simulink library "IOLib"  (R2016b)
settings: Solver=VariableStepAuto  StartTime=0.0  StopTime=10.0  RelTol=1e-3
undefined symbols (not defined in the file): EGPI, EGPO, EVADC
libraries: simulink x3
settings Model: Creator=Administrator  LastModifiedBy=Administrator

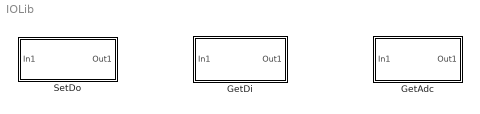
== system IOLib ==
  GetAdc : Subsystem  TreatAsAtomicUnit=on
      settings: OpenFcn=open_system([gcb,'/Enumerated Constant'],'mask');  RTWSystemCode=Inline
      mask Display:
      | tmpx = get_param([gcb,'/Enumerated Constant'],'Value');
      | disp(tmpx);
  GetDi : Subsystem  TreatAsAtomicUnit=on
      settings: OpenFcn=open_system([gcb,'/Enumerated Constant'],'mask');  PermitHierarchicalResolution=None  RTWSystemCode=Inline
      mask Display:
      | tmpx = get_param([gcb,'/Enumerated Constant'],'Value');
      | disp(tmpx);
  SetDo : Subsystem  TreatAsAtomicUnit=on
      settings: OpenFcn=open_system([gcb,'/Enumerated Constant'],'mask');  RTWSystemCode=Inline
      mask Display:
      | tmpx = get_param([gcb,'/Enumerated Constant'],'Value');
      | disp(tmpx);

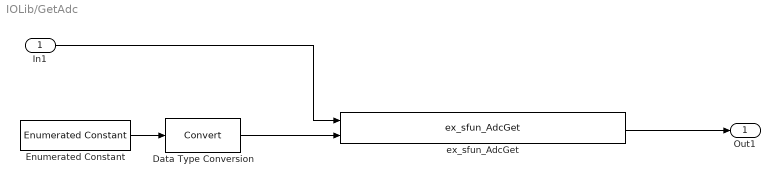
== system IOLib/GetAdc ==
  In1 : Inport
  Data Type Conversion : DataTypeConversion
  Enumerated Constant : simulink/Sources/Enumerated Constant  OutDataTypeStr=Enum: EVADC  Value=EVADC.UBR1  SampleTime=inf
  ex_sfun_AdcGet : S-Function  FunctionName=ex_sfun_AdcGet  SFunctionDeploymentMode=off  EnableBusSupport=off  mask(Legacy Function){SFunctionSpec=void AdcGetShell(uint16 u1, uint16 u2, uint16 y1[1]), ShowSpec=on}
      mask prompts: ShowSpec "Display function specification"
      mask help:
      | This block allows you to call the legacy functions specified by the following Legacy Code Tool definition:
      | def.SFunctionName = 'ex_sfun_AdcGet';
      | def.OutputFcnSpec = 'void AdcGetShell(uint16 u1, uint16 u2, uint16 y1[1])';
      | def.HeaderFiles = {'C2SfunShell.h', 'Platform_Types.h', 'LIB_Atan2.h', 'LIB_SinCosCalc.h', 'LIB_SqrtCalc.h'};
      | def.SourceFiles = {'C2SfunShell.c', 'LIB_Atan2.c', 'LIB_SinCosCalc.c', 'LIB_SqrtCalc.c'};
      mask Help: <p>This block was generated automatically by the Legacy Code Tool. For detailed help on this tool, call<a href="matlab:legacy_code('help')"> legacy_code('help')</a>.</p>
      mask Callback ShowSpec:
      | if strcmp(get_param(gcbh, 'ShowSpec'), 'on')
      |   set_param(gcbh, 'MaskDisplay', sprintf('fprintf(''%s'');', get_param(gcbh, 'SFunctionSpec')));
      | else
      |   set_param(gcbh, 'MaskDisplay', sprintf('fprintf(''%s'');', get_param(gcbh, 'FunctionName')));
      | end
      mask Display: fprintf('%s','void AdcGetShell(uint16 u1, uint16 u2, uint16 y1[1])');
  Out1 : Outport
  wires:
  Data Type Conversion/1 -> ex_sfun_AdcGet/2
  ex_sfun_AdcGet/1 -> Out1/1
  Enumerated Constant/1 -> Data Type Conversion/1
  In1/1 -> ex_sfun_AdcGet/1

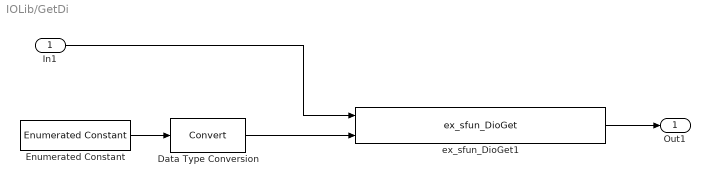
== system IOLib/GetDi ==
  In1 : Inport
  Data Type Conversion : DataTypeConversion
  Enumerated Constant : simulink/Sources/Enumerated Constant  OutDataTypeStr=Enum: EGPI  Value=EGPI.STL2ASCEN  SampleTime=inf
  ex_sfun_DioGet1 : S-Function  FunctionName=ex_sfun_DioGet  SFunctionDeploymentMode=off  EnableBusSupport=off  mask(Legacy Function){SFunctionSpec=void DioGetShell(boolean u1, uint16 u2, boolean y1[1]), ShowSpec=on}
      mask prompts: ShowSpec "Display function specification"
      mask help:
      | This block allows you to call the legacy functions specified by the following Legacy Code Tool definition:
      | def.SFunctionName = 'ex_sfun_DioGet';
      | def.OutputFcnSpec = 'void DioGetShell(boolean u1, uint16 u2, boolean y1[1])';
      | def.HeaderFiles = {'C2SfunShell.h', 'Platform_Types.h', 'LIB_Atan2.h', 'LIB_SinCosCalc.h', 'LIB_SqrtCalc.h'};
      | def.SourceFiles = {'C2SfunShell.c', 'LIB_Atan2.c', 'LIB_SinCosCalc.c', 'LIB_SqrtCalc.c'};
      mask Help: <p>This block was generated automatically by the Legacy Code Tool. For detailed help on this tool, call<a href="matlab:legacy_code('help')"> legacy_code('help')</a>.</p>
      mask Callback ShowSpec:
      | if strcmp(get_param(gcbh, 'ShowSpec'), 'on')
      |   set_param(gcbh, 'MaskDisplay', sprintf('fprintf(''%s'');', get_param(gcbh, 'SFunctionSpec')));
      | else
      |   set_param(gcbh, 'MaskDisplay', sprintf('fprintf(''%s'');', get_param(gcbh, 'FunctionName')));
      | end
      mask Display: fprintf('%s','void DioGetShell(boolean u1, uint16 u2, boolean y1[1])');
  Out1 : Outport
  wires:
  Enumerated Constant/1 -> Data Type Conversion/1
  Data Type Conversion/1 -> ex_sfun_DioGet1/2
  In1/1 -> ex_sfun_DioGet1/1
  ex_sfun_DioGet1/1 -> Out1/1

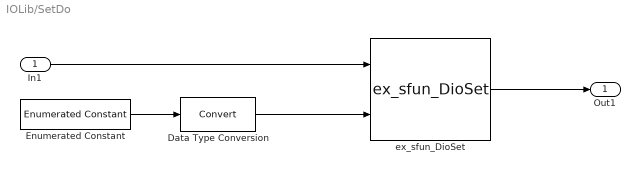
== system IOLib/SetDo ==
  In1 : Inport
  Data Type Conversion : DataTypeConversion
  Enumerated Constant : simulink/Sources/Enumerated Constant  OutDataTypeStr=Enum: EGPO  Value=EGPO.DISPWM  SampleTime=inf
  ex_sfun_DioSet : S-Function  FunctionName=ex_sfun_DioSet  SFunctionDeploymentMode=off  EnableBusSupport=off  mask(Legacy Function){SFunctionSpec=void DioSetShell(boolean u1, uint16 u2, boolean y1[1]), ShowSpec=on}
      mask prompts: ShowSpec "Display function specification"
      mask help:
      | This block allows you to call the legacy functions specified by the following Legacy Code Tool definition:
      | def.SFunctionName = 'ex_sfun_DioSet';
      | def.OutputFcnSpec = 'void DioSetShell(boolean u1, uint16 u2, boolean y1[1])';
      | def.HeaderFiles = {'C2SfunShell.h', 'Platform_Types.h', 'LIB_Atan2.h', 'LIB_SinCosCalc.h', 'LIB_SqrtCalc.h'};
      | def.SourceFiles = {'C2SfunShell.c', 'LIB_Atan2.c', 'LIB_SinCosCalc.c', 'LIB_SqrtCalc.c'};
      mask Help: <p>This block was generated automatically by the Legacy Code Tool. For detailed help on this tool, call<a href="matlab:legacy_code('help')"> legacy_code('help')</a>.</p>
      mask Callback ShowSpec:
      | if strcmp(get_param(gcbh, 'ShowSpec'), 'on')
      |   set_param(gcbh, 'MaskDisplay', sprintf('fprintf(''%s'');', get_param(gcbh, 'SFunctionSpec')));
      | else
      |   set_param(gcbh, 'MaskDisplay', sprintf('fprintf(''%s'');', get_param(gcbh, 'FunctionName')));
      | end
      mask Display: fprintf('%s','void DioSetShell(boolean u1, uint16 u2, boolean y1[1])');
  Out1 : Outport
  wires:
  Enumerated Constant/1 -> Data Type Conversion/1
  In1/1 -> ex_sfun_DioSet/1
  Data Type Conversion/1 -> ex_sfun_DioSet/2
  ex_sfun_DioSet/1 -> Out1/1
